simulink model "capitol5pb2"  (R2013a)
settings: Solver=ode45  StartTime=0.0  StopTime=300  RelTol=1e-3
undefined symbols (not defined in the file): des, gcbh
settings Model: Creator=user  LastModifiedBy=user

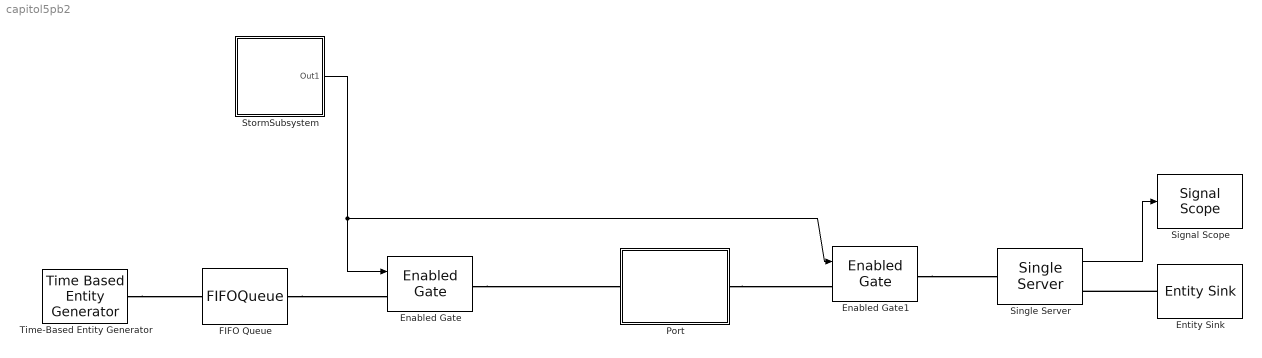
== system capitol5pb2 ==
  Enabled Gate : EnabledGate
  Enabled Gate1 : EnabledGate
  Entity Sink : EntitySink
  FIFO Queue : FIFOQueue
  "Port " : Subsystem
  Signal Scope : SignalScope  LoadFcn=des.scope.CallbackSupport('seLoadFcn',gcbh)  StartFcn=des.scope.CallbackSupport('seStartFcn',gcbh)  StopFcn=des.scope.CallbackSupport('seStopFcn',gcbh)
      settings: CopyFcn=des.scope.CallbackSupport('seCopyFcn',gcbh)  DeleteFcn=des.scope.CallbackSupport('seDeleteFcn',gcbh)  PreSaveFcn=des.scope.CallbackSupport('sePreSaveFcn',gcbh)  NameChangeFcn=des.scope.CallbackSupport('seNameChangeFcn',gcbh)  OpenFcn=des.scope.CallbackSupport('seOpenFcn',gcbh)
  Single Server : SingleServer  ServiceTime=0.5  StatNumberDeparted=on
  StormSubsystem : Subsystem
  Time-Based Entity Generator : TimeBasedEntityGenerator  Distribution=Uniform  Minimum=3  Maximum=5
  wires:
  StormSubsystem/1(Out1) -> Enabled Gate1/1, Enabled Gate/1
  Single Server/1 -> Signal Scope/1
  connections:
  Time-Based Entity Generator/RConn1 -- FIFO Queue/LConn1
  FIFO Queue/RConn1 -- Enabled Gate/LConn1
  Enabled Gate/RConn1 -- "Port "/LConn1
  "Port "/RConn1 -- Enabled Gate1/LConn1
  Enabled Gate1/RConn1 -- Single Server/LConn1
  Entity Sink/LConn1 -- Single Server/RConn1

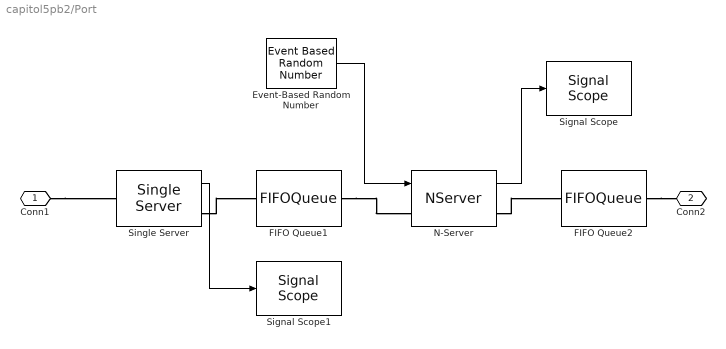
== system capitol5pb2/Port  ==
  Event-Based Random Number : EventBasedRandomNumber  Distribution=Uniform  minUnif=7  maxUnif=17
  FIFO Queue1 : FIFOQueue
  FIFO Queue2 : FIFOQueue
  N-Server : NServer  NumberOfServers=3  ServiceTimeFrom=Signal port t  StatNumberDeparted=on
  Signal Scope : SignalScope  LoadFcn=des.scope.CallbackSupport('seLoadFcn',gcbh)  StartFcn=des.scope.CallbackSupport('seStartFcn',gcbh)  StopFcn=des.scope.CallbackSupport('seStopFcn',gcbh)
      settings: CopyFcn=des.scope.CallbackSupport('seCopyFcn',gcbh)  DeleteFcn=des.scope.CallbackSupport('seDeleteFcn',gcbh)  PreSaveFcn=des.scope.CallbackSupport('sePreSaveFcn',gcbh)  NameChangeFcn=des.scope.CallbackSupport('seNameChangeFcn',gcbh)  OpenFcn=des.scope.CallbackSupport('seOpenFcn',gcbh)
  Signal Scope1 : SignalScope  LoadFcn=des.scope.CallbackSupport('seLoadFcn',gcbh)  StartFcn=des.scope.CallbackSupport('seStartFcn',gcbh)  StopFcn=des.scope.CallbackSupport('seStopFcn',gcbh)
      settings: CopyFcn=des.scope.CallbackSupport('seCopyFcn',gcbh)  DeleteFcn=des.scope.CallbackSupport('seDeleteFcn',gcbh)  PreSaveFcn=des.scope.CallbackSupport('sePreSaveFcn',gcbh)  NameChangeFcn=des.scope.CallbackSupport('seNameChangeFcn',gcbh)  OpenFcn=des.scope.CallbackSupport('seOpenFcn',gcbh)
  Single Server : SingleServer  StatNumberDeparted=on
  Conn1 : PMIOPort  Port=1  Side=Left
  Conn2 : PMIOPort  Port=2  Side=Right
  wires:
  Event-Based Random Number/1 -> N-Server/1
  Single Server/1 -> Signal Scope1/1
  N-Server/1 -> Signal Scope/1
  connections:
  FIFO Queue1/RConn1 -- N-Server/LConn1
  Conn1/RConn1 -- Single Server/LConn1
  Single Server/RConn1 -- FIFO Queue1/LConn1
  FIFO Queue2/RConn1 -- Conn2/RConn1
  N-Server/RConn1 -- FIFO Queue2/LConn1

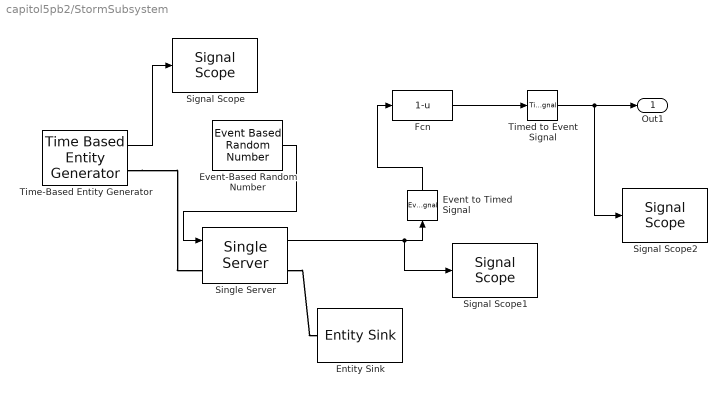
== system capitol5pb2/StormSubsystem ==
  Entity Sink : EntitySink
  Event to Timed Signal : EventToTimedSignal
  Event-Based Random Number : EventBasedRandomNumber  Distribution=Uniform  minUnif=2  maxUnif=6
  Fcn : Fcn  Expr=1-u
  Signal Scope : SignalScope  LoadFcn=des.scope.CallbackSupport('seLoadFcn',gcbh)  StartFcn=des.scope.CallbackSupport('seStartFcn',gcbh)  StopFcn=des.scope.CallbackSupport('seStopFcn',gcbh)
      settings: CopyFcn=des.scope.CallbackSupport('seCopyFcn',gcbh)  DeleteFcn=des.scope.CallbackSupport('seDeleteFcn',gcbh)  PreSaveFcn=des.scope.CallbackSupport('sePreSaveFcn',gcbh)  NameChangeFcn=des.scope.CallbackSupport('seNameChangeFcn',gcbh)  OpenFcn=des.scope.CallbackSupport('seOpenFcn',gcbh)
  Signal Scope1 : SignalScope  LoadFcn=des.scope.CallbackSupport('seLoadFcn',gcbh)  StartFcn=des.scope.CallbackSupport('seStartFcn',gcbh)  StopFcn=des.scope.CallbackSupport('seStopFcn',gcbh)
      settings: CopyFcn=des.scope.CallbackSupport('seCopyFcn',gcbh)  DeleteFcn=des.scope.CallbackSupport('seDeleteFcn',gcbh)  PreSaveFcn=des.scope.CallbackSupport('sePreSaveFcn',gcbh)  NameChangeFcn=des.scope.CallbackSupport('seNameChangeFcn',gcbh)  OpenFcn=des.scope.CallbackSupport('seOpenFcn',gcbh)
  Signal Scope2 : SignalScope  LoadFcn=des.scope.CallbackSupport('seLoadFcn',gcbh)  StartFcn=des.scope.CallbackSupport('seStartFcn',gcbh)  StopFcn=des.scope.CallbackSupport('seStopFcn',gcbh)
      settings: CopyFcn=des.scope.CallbackSupport('seCopyFcn',gcbh)  DeleteFcn=des.scope.CallbackSupport('seDeleteFcn',gcbh)  PreSaveFcn=des.scope.CallbackSupport('sePreSaveFcn',gcbh)  NameChangeFcn=des.scope.CallbackSupport('seNameChangeFcn',gcbh)  OpenFcn=des.scope.CallbackSupport('seOpenFcn',gcbh)
  Single Server : SingleServer  ServiceTimeFrom=Signal port t  StatNumberInBlock=on
      settings: OutputPortMap=o1
  Time-Based Entity Generator : TimeBasedEntityGenerator  Distribution=Uniform  Minimum=44  Maximum=52  Mean=0.5  StatNumberDeparted=on
  Timed to Event Signal : TimedToEventSignal
  Out1 : Outport
  wires:
  Time-Based Entity Generator/1 -> Signal Scope/1
  Event-Based Random Number/1 -> Single Server/1
  Event to Timed Signal/1 -> Fcn/1
  Single Server/1 -> Signal Scope1/1, Event to Timed Signal/1
  Fcn/1 -> Timed to Event Signal/1
  Timed to Event Signal/1 -> Out1/1, Signal Scope2/1
  connections:
  Time-Based Entity Generator/RConn1 -- Single Server/LConn1
  Single Server/RConn1 -- Entity Sink/LConn1
